simulink model "FM_recv"  (R2019a)
settings: Solver=VariableStepAuto  StartTime=0.0  StopTime=0.05  FixedStep=8e-9  RelTol=1e-3
libraries: dspfdesign x5, commanapbnd3 x3
settings Model: Creator=Wunyje  LastModifiedBy=Wunyje

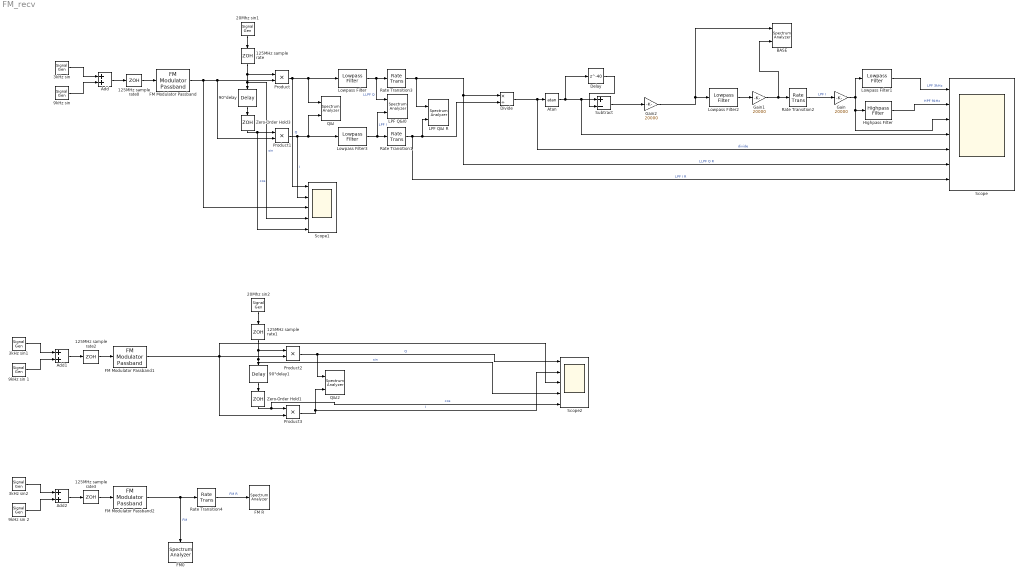
== system FM_recv ==
  125MHz sample rate{,0,2..3} (4 alike) : ZeroOrderHold  SampleTime=8e-9
  125MHz sample rate1 : ZeroOrderHold  SampleTime=8E-9
  20Mhz sin1 : SignalGenerator  Frequency=20e6
  20Mhz sin2 : SignalGenerator  Frequency=20e6
  3kHz sin : SignalGenerator  Frequency=3000
  3kHz sin1 : SignalGenerator  Frequency=3000
  3kHz sin2 : SignalGenerator  Frequency=3000
  90°delay : TransportDelay  DelayTime=12.5e-9
  90°delay1 : TransportDelay  DelayTime=12.5e-9
  "9kHz sin " : SignalGenerator  Frequency=9000
  9kHz sin 1 : SignalGenerator  Frequency=9000
  9kHz sin 2 : SignalGenerator  Frequency=9000
  Add : Sum
  Add1 : Sum
  Add2 : Sum
  Atan : Trigonometry  Operator=atan
  BASE : SpectrumAnalyzer  NumInputPorts=2
  Delay : Delay  DelayLength=40  InitialCondition=0
  Divide : Product  Inputs=*/
  FM Modulator Passband : commanapbnd3/FM Modulator Passband  Fc=20e6  Ph=0  Kc=1e6
      settings: SourceProductName=Communications Toolbox  SourceProductBaseCode=CM
  FM Modulator Passband1 : commanapbnd3/FM Modulator Passband  Fc=20e6  Ph=0  Kc=1E6
      settings: SourceProductName=Communications Toolbox  SourceProductBaseCode=CM
  FM Modulator Passband2 : commanapbnd3/FM Modulator Passband  Fc=20e6  Ph=0  Kc=1E6
      settings: SourceProductName=Communications Toolbox  SourceProductBaseCode=CM
  FM R : SpectrumAnalyzer
  FM0 : SpectrumAnalyzer
  Gain : Gain  Gain=20000
  Gain1 : Gain  Gain=20000
  Gain2 : Gain  Gain=20000
  Highpass Filter : dspfdesign/Highpass Filter  FilterType=FIR  DesignForMinimumOrder=on  FilterOrder=50  StopbandFrequency=4e3  PassbandFrequency=6e3  StopbandAttenuation=80  PassbandRipple=0.1  InheritSampleRate=on  SampleRate=50e3  SimulateUsing=Interpreted execution  roundingMode=Floor  coeffsDataTypeStr=fixdt(1,16)
      settings: SourceProductName=DSP System Toolbox
  LPF Q&I R : SpectrumAnalyzer  NumInputPorts=2
  LPF Q&I0 : SpectrumAnalyzer  NumInputPorts=2
  Lowpass Filter : dspfdesign/Lowpass Filter  FilterType=FIR  DesignForMinimumOrder=on  FilterOrder=50  PassbandFrequency=30e6  StopbandFrequency=35e6  PassbandRipple=0.01  StopbandAttenuation=90  InheritSampleRate=off  SampleRate=125e6  SimulateUsing=Interpreted execution  roundingMode=Floor  coeffsDataTypeStr=fixdt(1,16)
  Lowpass Filter1 : dspfdesign/Lowpass Filter  FilterType=FIR  DesignForMinimumOrder=on  FilterOrder=50  PassbandFrequency=5e3  StopbandFrequency=7e3  PassbandRipple=0.1  StopbandAttenuation=80  InheritSampleRate=on  SampleRate=200e3  SimulateUsing=Interpreted execution  roundingMode=Floor  coeffsDataTypeStr=fixdt(1,16)
  Lowpass Filter2 : dspfdesign/Lowpass Filter  FilterType=FIR  DesignForMinimumOrder=on  FilterOrder=50  PassbandFrequency=150e3  StopbandFrequency=190e3  PassbandRipple=0.1  StopbandAttenuation=60  InheritSampleRate=off  SampleRate=25E6  SimulateUsing=Interpreted execution  roundingMode=Floor  coeffsDataTypeStr=fixdt(1,16)
  Lowpass Filter3 : dspfdesign/Lowpass Filter  FilterType=FIR  DesignForMinimumOrder=on  FilterOrder=50  PassbandFrequency=30e6  StopbandFrequency=35e6  PassbandRipple=0.01  StopbandAttenuation=90  InheritSampleRate=off  SampleRate=125e6  SimulateUsing=Interpreted execution  roundingMode=Floor  coeffsDataTypeStr=fixdt(1,16)
  Product{,1..3} (4 alike) : Product
  Q&I : SpectrumAnalyzer  NumInputPorts=2
  Q&I2 : SpectrumAnalyzer  NumInputPorts=2
  Rate Transition1 : RateTransition  OutPortSampleTimeOpt=Multiple of input port sample time  OutPortSampleTimeMultiple=25
  Rate Transition2 : RateTransition  OutPortSampleTimeOpt=Multiple of input port sample time  OutPortSampleTimeMultiple=50
  Rate Transition3 : RateTransition  OutPortSampleTimeOpt=Multiple of input port sample time  OutPortSampleTimeMultiple=25
  Rate Transition4 : RateTransition  OutPortSampleTimeOpt=Multiple of input port sample time  OutPortSampleTimeMultiple=2
  Scope : Scope  NumInputPorts=7
  Scope1 : Scope  NumInputPorts=5
  Scope2 : Scope  NumInputPorts=5
  Subtract : Sum  Inputs=+-
  Zero-Order Hold1 : ZeroOrderHold  SampleTime=8E-9
  Zero-Order Hold3 : ZeroOrderHold  SampleTime=8e-9
  wires:
  90°delay/1 -> Zero-Order Hold3/1
  Zero-Order Hold3/1 -> Scope1/5, Product1/1  "cos"
  Product/1 -> Q&I/1, Lowpass Filter/1, Scope1/1  "Q"
  20Mhz sin1/1 -> 125MHz sample rate/1
  Subtract/1 -> Gain2/1
  Atan/1 -> Delay/1, Subtract/1, Scope/4
  Gain/1 -> Lowpass Filter1/1, Scope/3, Highpass Filter/1
  Add/1 -> 125MHz sample rate0/1
  Highpass Filter/1 -> Scope/2  "HPF 9kHz"
  Product1/1 -> Scope1/2, Lowpass Filter3/1, Q&I/2  "I"
  FM Modulator Passband/1 -> Scope1/3, Product/2, Product1/2
  Lowpass Filter/1 -> LPF Q&I0/1, Rate Transition3/1  "LLPF Q"
  "9kHz sin "/1 -> Add/2
  Delay/1 -> Subtract/2
  125MHz sample rate/1 -> Scope1/4, 90°delay/1, Product/1  "sin"
  125MHz sample rate0/1 -> FM Modulator Passband/1
  Lowpass Filter3/1 -> Rate Transition1/1, LPF Q&I0/2  "LPF I"
  3kHz sin/1 -> Add/1
  Rate Transition2/1 -> Gain/1  "LPF I"
  Lowpass Filter2/1 -> Gain1/1
  Divide/1 -> Scope/5, Atan/1  "divide"
  Lowpass Filter1/1 -> Scope/1  "LPF 3kHz"
  Rate Transition1/1 -> LPF Q&I R/2, Divide/2, Scope/7  "LPF I R"
  Rate Transition3/1 -> Scope/6, Divide/1, LPF Q&I R/1  "LLPF Q R"
  Gain1/1 -> BASE/2, Rate Transition2/1
  9kHz sin 1/1 -> Add1/2
  125MHz sample rate1/1 -> Scope2/4, 90°delay1/1, Product2/1  "sin"
  90°delay1/1 -> Zero-Order Hold1/1
  20Mhz sin2/1 -> 125MHz sample rate1/1
  3kHz sin1/1 -> Add1/1
  Zero-Order Hold1/1 -> Scope2/5, Product3/1  "cos"
  FM Modulator Passband1/1 -> Product2/2, Product3/2, Scope2/3
  125MHz sample rate2/1 -> FM Modulator Passband1/1
  Product3/1 -> Scope2/2, Q&I2/2  "I"
  Add1/1 -> 125MHz sample rate2/1
  Product2/1 -> Scope2/1, Q&I2/1  "Q"
  Gain2/1 -> BASE/1, Lowpass Filter2/1
  Add2/1 -> 125MHz sample rate3/1
  125MHz sample rate3/1 -> FM Modulator Passband2/1
  3kHz sin2/1 -> Add2/1
  FM Modulator Passband2/1 -> Rate Transition4/1, FM0/1  "FM"
  9kHz sin 2/1 -> Add2/2
  Rate Transition4/1 -> FM R/1  "FM R"
